simulink model "PI Controller Vector Controlled IM Drive"  (R2020b)
settings: Solver=ode4  StartTime=0.0  StopTime=5  RelTol=1e-3
InitFcn:
  | %clear;
  | %clc;
  | 
  | %Motor Parameters
  | r1 = 1.405;
  | l1  = 0.005839;
  | r2 = 1.395;
  | l2 = 0.005839;
  | Lm = 0.1722;
  | J = 0.0131;
  | 
  | %Motor Rated Values
  | Vrat = 400;
  | frat = 50;
  | 
  | x1 = 2*pi*frat*l1;
  | x2 = 2*pi*frat*l2;
  | Xm = 2*pi*frat*Lm;
  | Prat = 4*1000;
  | Nrat = 1430;
  | P = 4;
  | Ns = 120*frat/P;
  | nrat = Nrat*2*pi/60;
  | ns = Ns*2*pi/60;
  | srat = (Ns-Nrat)/Ns;
  | 
  | E1 = Vrat/sqrt(3); %phase voltage
  | IL = E1/( (r1 + (1i*x1) ) + ( ( (1i*x2) +(r2/srat) )*1i*Xm / ( (1i*Xm) + (1i*x2) + (r2/srat) ) ) );
  | E2 = E1 - (IL*(r1 + (1i*x1) ) );
  | Trat = (3/(ns))*srat*abs(E2)*abs(E2)*r2/((r2*r2) + (srat*srat*x2*x2));
  | %Trat = Prat/nrat;
  | 
  | %System Variables
  | Tsys = (1e-6);
  | Ts = (100e-6);
  | freq = 50;
  | ws = freq*2*pi;
  | 
  | m=1*freq/50;
  | %m = 1 * (freq/50);
  | Vbus = (400*sqrt(2)*2/sqrt(3)) / (1.15);
  | 
  | Vref = (Vbus*sqrt(3)/2) * m;
  | delay = Ts/Tsys;
  | 
  | % Motor Starting Parameters
  | inc_time = 0.1;
  | 
  | %Motor Loading time
  | load_time = 0;
  | 
  | %No. of Hybrid Zones
  | numzones = 3;
  | 
  | %Load ML model Weights
  | 
  | W1R_s1 = readmatrix('Regression Weights\W1_subnet1_tmp_odd_90.xlsx');
  | b1R_s1 = readmatrix('Regression Weights\b1_subnet1_tmp_odd_90.xlsx');
  | W1R_s2 = readmatrix('Regression Weights\W1_subnet2_tmp_odd_90.xlsx');
  | b1R_s2 = readmatrix('Regression Weights\b1_subnet2_tmp_odd_90.xlsx');
  | ... (+35 lines)
undefined symbols (not defined in the file): DiscIntNeverNeededParam
libraries: powerlib x21, simulink x19, pid_lib x4, powerlib_meascontrol x4, simulink_extras x2
(part 2 of 3)

== system PI Controller Vector Controlled IM Drive/Space Vector PWM based VSI 1/Gating Pulse Generator/Gate Pulse Generator for 2721 Sequence ==
  "S1, S3, S5, sector" : Inport
  AND{,1..5} (6 alike) : Logic  IconShape=distinctive  AllPortsSameDT=off  OutDataTypeStr=boolean
  Constant : Constant  Value=2
  Data Type Conversion : DataTypeConversion
  Demux : Demux
  For Even Sector : Subsystem
  For Odd Sector : Subsystem
  Mod : Math  Operator=mod  SaturateOnIntegerOverflow=on
  Mux : Mux  Inputs=3
  NOT : Logic  Operator=NOT  IconShape=distinctive  AllPortsSameDT=off  OutDataTypeStr=boolean
  OR : Logic  Operator=OR  IconShape=distinctive  AllPortsSameDT=off  OutDataTypeStr=boolean
  OR1 : Logic  Operator=OR  IconShape=distinctive  AllPortsSameDT=off  OutDataTypeStr=boolean
  OR2 : Logic  Operator=OR  IconShape=distinctive  AllPortsSameDT=off  OutDataTypeStr=boolean
  Scope1 : Scope  NumInputPorts=4
  Gate 1 Pulse : Outport
  Gate 3 Pulse : Outport  Port=2
  Gate 5 Pulse : Outport  Port=3
  wires:
  For Odd Sector/3(Gate 5 Pulse) -> AND5/1
  For Odd Sector/1(Gate 1 Pulse) -> AND3/1
  For Even Sector/3(Gate 5 Pulse) -> AND2/1
  OR2/1 -> Scope1/3, Gate 5 Pulse/1
  For Even Sector/2(Gate 3 Pulse) -> AND1/1
  OR1/1 -> Scope1/2, Gate 3 Pulse/1
  Demux/3 -> Mux/3
  AND4/1 -> OR1/1
  OR/1 -> Scope1/1, Gate 1 Pulse/1
  AND5/1 -> OR2/1
  Demux/2 -> Mux/2
  For Odd Sector/2(Gate 3 Pulse) -> AND4/1
  AND1/1 -> OR1/2
  AND/1 -> OR/2
  Mod/1 -> Data Type Conversion/1
  Data Type Conversion/1 -> AND3/2, AND4/2, AND5/2, NOT/1
  AND2/1 -> OR2/2
  "S1, S3, S5, sector"/1 -> Demux/1
  AND3/1 -> OR/1
  Demux/4 -> Scope1/4, Mod/1
  Demux/1 -> Mux/1
  Mux/1 -> For Even Sector/1("S1, S3, S5"), For Odd Sector/1("S1, S3, S1")
  Constant/1 -> Mod/2
  NOT/1 -> AND/2, AND1/2, AND2/2
  For Even Sector/1(Gate 1 Pulse) -> AND/1

== system PI Controller Vector Controlled IM Drive/Space Vector PWM based VSI 1/Gating Pulse Generator/Gate Pulse Generator for 7212 Sequence ==
  "S1, S3, S5, sector" : Inport
  AND{,1..5} (6 alike) : Logic  IconShape=distinctive  AllPortsSameDT=off  OutDataTypeStr=boolean
  Constant : Constant  Value=2
  Data Type Conversion : DataTypeConversion
  Demux : Demux
  For Even Sector : Subsystem
  For Odd Sector : Subsystem
  Mod : Math  Operator=mod  SaturateOnIntegerOverflow=on
  Mux : Mux  Inputs=3
  NOT : Logic  Operator=NOT  IconShape=distinctive  AllPortsSameDT=off  OutDataTypeStr=boolean
  OR : Logic  Operator=OR  IconShape=distinctive  AllPortsSameDT=off  OutDataTypeStr=boolean
  OR1 : Logic  Operator=OR  IconShape=distinctive  AllPortsSameDT=off  OutDataTypeStr=boolean
  OR2 : Logic  Operator=OR  IconShape=distinctive  AllPortsSameDT=off  OutDataTypeStr=boolean
  Scope1 : Scope  NumInputPorts=4
  Gate 1 Pulse : Outport
  Gate 3 Pulse : Outport  Port=2
  Gate 5 Pulse : Outport  Port=3
  wires:
  For Odd Sector/3(Gate 5 Pulse) -> AND5/1
  For Odd Sector/1(Gate 1 Pulse) -> AND3/1
  For Even Sector/3(Gate 5 Pulse) -> AND2/1
  For Even Sector/2(Gate 3 Pulse) -> AND1/1
  OR2/1 -> Scope1/3, Gate 5 Pulse/1
  OR1/1 -> Scope1/2, Gate 3 Pulse/1
  Demux/3 -> Mux/3
  For Even Sector/1(Gate 1 Pulse) -> AND/1
  AND4/1 -> OR1/1
  OR/1 -> Scope1/1, Gate 1 Pulse/1
  AND5/1 -> OR2/1
  Demux/2 -> Mux/2
  AND1/1 -> OR1/2
  AND/1 -> OR/2
  Mod/1 -> Data Type Conversion/1
  Demux/4 -> Scope1/4, Mod/1
  Data Type Conversion/1 -> AND3/2, AND4/2, AND5/2, NOT/1
  AND2/1 -> OR2/2
  Demux/1 -> Mux/1
  Mux/1 -> For Even Sector/1("S1, S3, S1"), For Odd Sector/1("S1, S3, S5")
  Constant/1 -> Mod/2
  NOT/1 -> AND/2, AND1/2, AND2/2
  For Odd Sector/2(Gate 3 Pulse) -> AND4/1
  "S1, S3, S5, sector"/1 -> Demux/1
  AND3/1 -> OR/1

== system PI Controller Vector Controlled IM Drive/Space Vector PWM based VSI 1/Switching Times and Sector/Angle Calculation1 ==
  freq : Inport
  Delay : Delay  DelayLength=1  InitialCondition=0  UseCircularBuffer=on
  Gain1 : Gain  Gain=Tsys
  MATLAB Function : MATLAB Function  TreatAsAtomicUnit=on
  Scope : Scope
  Zero-Order Hold : ZeroOrderHold  SampleTime=Ts
  w : Gain  Gain=2*pi
  Angle : Outport
  tag scope: wt=global
  wires:
  freq/1 -> w/1, Scope/1
  Gain1/1 -> MATLAB Function/2(wTs)
  Zero-Order Hold/1 -> Angle/1
  Delay/1 -> MATLAB Function/1(wold)
  MATLAB Function/1(wnew) -> Delay/1, Zero-Order Hold/1, [wt]
  w/1 -> Gain1/1

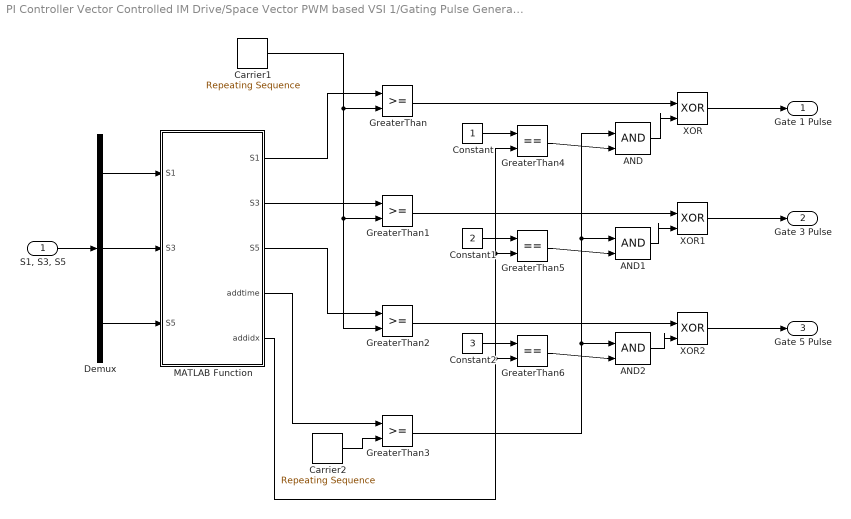
== system PI Controller Vector Controlled IM Drive/Space Vector PWM based VSI 1/Gating Pulse Generator/Gate Pulse Generator for 0121 Sequence/For Even Sector ==
  "S1, S3, S5" : Inport
  AND : Logic  IconShape=distinctive  AllPortsSameDT=off  OutDataTypeStr=boolean
  AND1 : Logic  IconShape=distinctive  AllPortsSameDT=off  OutDataTypeStr=boolean
  AND2 : Logic  IconShape=distinctive  AllPortsSameDT=off  OutDataTypeStr=boolean
  Carrier1 : simulink/Sources/Repeating Sequence  rep_seq_t=[0 Ts/2 Ts]  rep_seq_y=[0 Ts-(1e-16) 0]
  Carrier2 : simulink/Sources/Repeating Sequence  rep_seq_t=[0 Ts/2 Ts]  rep_seq_y=[Ts-(1e-16) 0 Ts-(1e-16)]
  Constant : Constant
  Constant1 : Constant  Value=2
  Constant2 : Constant  Value=3
  Demux : Demux  Outputs=3
  GreaterThan{,1..3} (4 alike) : RelationalOperator  OutDataTypeStr=boolean  RndMeth=Simplest
  GreaterThan4 : RelationalOperator  Operator===  OutDataTypeStr=boolean  RndMeth=Simplest
  GreaterThan5 : RelationalOperator  Operator===  OutDataTypeStr=boolean  RndMeth=Simplest
  GreaterThan6 : RelationalOperator  Operator===  OutDataTypeStr=boolean  RndMeth=Simplest
  MATLAB Function : MATLAB Function  TreatAsAtomicUnit=on
  XOR : Logic  Operator=XOR  IconShape=distinctive  AllPortsSameDT=off  OutDataTypeStr=boolean
  XOR1 : Logic  Operator=XOR  IconShape=distinctive  AllPortsSameDT=off  OutDataTypeStr=boolean
  XOR2 : Logic  Operator=XOR  IconShape=distinctive  AllPortsSameDT=off  OutDataTypeStr=boolean
  Gate 1 Pulse : Outport
  Gate 3 Pulse : Outport  Port=2
  Gate 5 Pulse : Outport  Port=3
  wires:
  Demux/3 -> MATLAB Function/3("S5 ")
  Demux/1 -> MATLAB Function/1("S1 ")
  "S1, S3, S5"/1 -> Demux/1
  Demux/2 -> MATLAB Function/2("S3 ")
  MATLAB Function/5(addidx) -> GreaterThan6/2, GreaterThan5/2, GreaterThan4/2
  Constant1/1 -> GreaterThan5/1
  Constant/1 -> GreaterThan4/1
  XOR1/1 -> Gate 3 Pulse/1
  GreaterThan6/1 -> AND2/2
  Constant2/1 -> GreaterThan6/1
  GreaterThan5/1 -> AND1/2
  AND/1 -> XOR/2
  AND2/1 -> XOR2/2
  GreaterThan2/1 -> XOR2/1
  MATLAB Function/1(S1) -> GreaterThan/1
  GreaterThan/1 -> XOR/1
  MATLAB Function/4(addtime) -> GreaterThan3/1
  GreaterThan4/1 -> AND/2
  XOR2/1 -> Gate 5 Pulse/1
  GreaterThan3/1 -> AND/1, AND1/1, AND2/1
  AND1/1 -> XOR1/2
  MATLAB Function/3(S5) -> GreaterThan2/1
  MATLAB Function/2(S3) -> GreaterThan1/1
  XOR/1 -> Gate 1 Pulse/1
  Carrier1/1 -> GreaterThan/2, GreaterThan1/2, GreaterThan2/2
  GreaterThan1/1 -> XOR1/1
  Carrier2/1 -> GreaterThan3/2

== system PI Controller Vector Controlled IM Drive/Space Vector PWM based VSI 1/Gating Pulse Generator/Gate Pulse Generator for 0121 Sequence/For Odd Sector ==
  "S1, S3, S5" : Inport
  AND : Logic  IconShape=distinctive  AllPortsSameDT=off  OutDataTypeStr=boolean
  AND1 : Logic  IconShape=distinctive  AllPortsSameDT=off  OutDataTypeStr=boolean
  AND2 : Logic  IconShape=distinctive  AllPortsSameDT=off  OutDataTypeStr=boolean
  Carrier1 : simulink/Sources/Repeating Sequence  rep_seq_t=[0 Ts/2 Ts]  rep_seq_y=[Ts-(1e-16) 0 Ts-(1e-16)]
  Constant : Constant
  Constant1 : Constant  Value=2
  Constant2 : Constant  Value=3
  Demux : Demux  Outputs=3
  GreaterThan{,1..3} (4 alike) : RelationalOperator  OutDataTypeStr=boolean  RndMeth=Simplest
  GreaterThan4 : RelationalOperator  Operator===  OutDataTypeStr=boolean  RndMeth=Simplest
  GreaterThan5 : RelationalOperator  Operator===  OutDataTypeStr=boolean  RndMeth=Simplest
  GreaterThan6 : RelationalOperator  Operator===  OutDataTypeStr=boolean  RndMeth=Simplest
  MATLAB Function : MATLAB Function  TreatAsAtomicUnit=on
  XOR : Logic  Operator=XOR  IconShape=distinctive  AllPortsSameDT=off  OutDataTypeStr=boolean
  XOR1 : Logic  Operator=XOR  IconShape=distinctive  AllPortsSameDT=off  OutDataTypeStr=boolean
  XOR2 : Logic  Operator=XOR  IconShape=distinctive  AllPortsSameDT=off  OutDataTypeStr=boolean
  Gate 1 Pulse : Outport
  Gate 3 Pulse : Outport  Port=2
  Gate 5 Pulse : Outport  Port=3
  wires:
  "S1, S3, S5"/1 -> Demux/1
  Demux/1 -> MATLAB Function/1("S1 ")
  Demux/2 -> MATLAB Function/2("S3 ")
  Demux/3 -> MATLAB Function/3("S5 ")
  MATLAB Function/1(S1) -> GreaterThan/1
  Carrier1/1 -> GreaterThan/2, GreaterThan1/2, GreaterThan3/2, GreaterThan2/2
  MATLAB Function/2(S3) -> GreaterThan1/1
  MATLAB Function/3(S5) -> GreaterThan2/1
  MATLAB Function/4(subtime) -> GreaterThan3/1
  MATLAB Function/5(subidx) -> GreaterThan6/2, GreaterThan5/2, GreaterThan4/2
  Constant/1 -> GreaterThan4/1
  Constant1/1 -> GreaterThan5/1
  Constant2/1 -> GreaterThan6/1
  GreaterThan4/1 -> AND/2
  GreaterThan5/1 -> AND1/2
  GreaterThan6/1 -> AND2/2
  GreaterThan3/1 -> AND/1, AND1/1, AND2/1
  AND/1 -> XOR/2
  GreaterThan/1 -> XOR/1
  GreaterThan1/1 -> XOR1/1
  AND1/1 -> XOR1/2
  GreaterThan2/1 -> XOR2/1
  AND2/1 -> XOR2/2
  XOR/1 -> Gate 1 Pulse/1
  XOR1/1 -> Gate 3 Pulse/1
  XOR2/1 -> Gate 5 Pulse/1

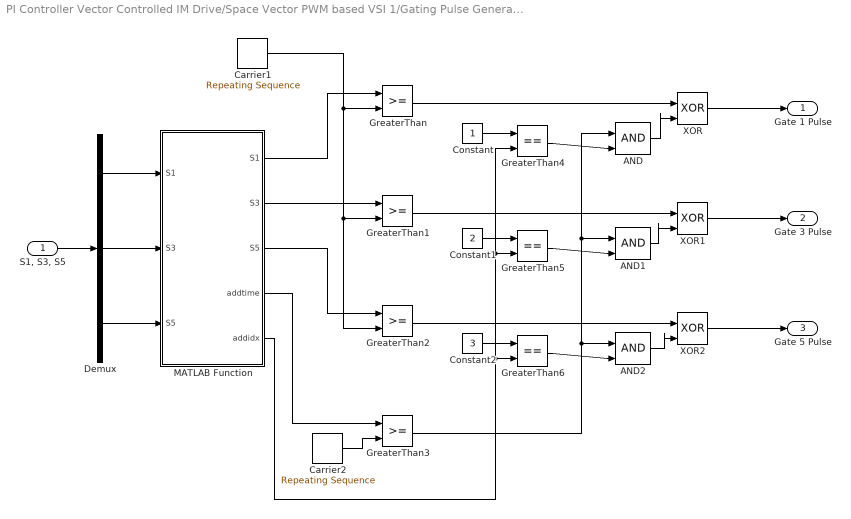
== system PI Controller Vector Controlled IM Drive/Space Vector PWM based VSI 1/Gating Pulse Generator/Gate Pulse Generator for 0127 Sequence 1/For Even Sector ==
  "S1, S3, S5" : Inport
  AND : Logic  IconShape=distinctive  AllPortsSameDT=off  OutDataTypeStr=boolean
  AND1 : Logic  IconShape=distinctive  AllPortsSameDT=off  OutDataTypeStr=boolean
  AND2 : Logic  IconShape=distinctive  AllPortsSameDT=off  OutDataTypeStr=boolean
  Carrier1 : simulink/Sources/Repeating Sequence  rep_seq_t=[0 Ts/2 Ts]  rep_seq_y=[Ts-(1e-16) 0 Ts-(1e-16)]
  Carrier2 : simulink/Sources/Repeating Sequence  rep_seq_t=[0 Ts/2 Ts]  rep_seq_y=[0 Ts-(1e-16) 0]
  Constant : Constant
  Constant1 : Constant  Value=2
  Constant2 : Constant  Value=3
  Demux : Demux  Outputs=3
  GreaterThan{,1..3} (4 alike) : RelationalOperator  OutDataTypeStr=boolean  RndMeth=Simplest
  GreaterThan4 : RelationalOperator  Operator===  OutDataTypeStr=boolean  RndMeth=Simplest
  GreaterThan5 : RelationalOperator  Operator===  OutDataTypeStr=boolean  RndMeth=Simplest
  GreaterThan6 : RelationalOperator  Operator===  OutDataTypeStr=boolean  RndMeth=Simplest
  MATLAB Function : MATLAB Function  TreatAsAtomicUnit=on
  XOR : Logic  Operator=XOR  IconShape=distinctive  AllPortsSameDT=off  OutDataTypeStr=boolean
  XOR1 : Logic  Operator=XOR  IconShape=distinctive  AllPortsSameDT=off  OutDataTypeStr=boolean
  XOR2 : Logic  Operator=XOR  IconShape=distinctive  AllPortsSameDT=off  OutDataTypeStr=boolean
  Gate 1 Pulse : Outport
  Gate 3 Pulse : Outport  Port=2
  Gate 5 Pulse : Outport  Port=3
  wires:
  AND/1 -> XOR/2
  GreaterThan2/1 -> XOR2/1
  "S1, S3, S5"/1 -> Demux/1
  MATLAB Function/1(S1) -> GreaterThan/1
  Demux/1 -> MATLAB Function/1("S1 ")
  Demux/2 -> MATLAB Function/2("S3 ")
  Demux/3 -> MATLAB Function/3("S5 ")
  Carrier2/1 -> GreaterThan3/2
  XOR2/1 -> Gate 5 Pulse/1
  GreaterThan6/1 -> AND2/2
  GreaterThan1/1 -> XOR1/1
  GreaterThan3/1 -> AND/1, AND1/1, AND2/1
  GreaterThan4/1 -> AND/2
  Constant2/1 -> GreaterThan6/1
  AND1/1 -> XOR1/2
  MATLAB Function/2(S3) -> GreaterThan1/1
  MATLAB Function/4(addtime) -> GreaterThan3/1
  XOR/1 -> Gate 1 Pulse/1
  Carrier1/1 -> GreaterThan/2, GreaterThan1/2, GreaterThan2/2
  Constant/1 -> GreaterThan4/1
  MATLAB Function/5(addidx) -> GreaterThan6/2, GreaterThan5/2, GreaterThan4/2
  GreaterThan5/1 -> AND1/2
  GreaterThan/1 -> XOR/1
  XOR1/1 -> Gate 3 Pulse/1
  MATLAB Function/3(S5) -> GreaterThan2/1
  AND2/1 -> XOR2/2
  Constant1/1 -> GreaterThan5/1

== system PI Controller Vector Controlled IM Drive/Space Vector PWM based VSI 1/Gating Pulse Generator/Gate Pulse Generator for 0127 Sequence 1/For Odd Sector ==
  "S1, S3, S1" : Inport
  AND3 : Logic  IconShape=distinctive  AllPortsSameDT=off  OutDataTypeStr=boolean
  AND4 : Logic  IconShape=distinctive  AllPortsSameDT=off  OutDataTypeStr=boolean
  AND5 : Logic  IconShape=distinctive  AllPortsSameDT=off  OutDataTypeStr=boolean
  Carrier3 : simulink/Sources/Repeating Sequence  rep_seq_t=[0 Ts/2 Ts]  rep_seq_y=[0 Ts-(1e-16) 0]
  Constant3 : Constant
  Constant4 : Constant  Value=2
  Constant5 : Constant  Value=3
  Demux1 : Demux  Outputs=3
  GreaterThan{7..10} (4 alike) : RelationalOperator  OutDataTypeStr=boolean  RndMeth=Simplest
  GreaterThan11 : RelationalOperator  Operator===  OutDataTypeStr=boolean  RndMeth=Simplest
  GreaterThan12 : RelationalOperator  Operator===  OutDataTypeStr=boolean  RndMeth=Simplest
  GreaterThan13 : RelationalOperator  Operator===  OutDataTypeStr=boolean  RndMeth=Simplest
  MATLAB Function1 : MATLAB Function  TreatAsAtomicUnit=on
  XOR3 : Logic  Operator=XOR  IconShape=distinctive  AllPortsSameDT=off  OutDataTypeStr=boolean
  XOR4 : Logic  Operator=XOR  IconShape=distinctive  AllPortsSameDT=off  OutDataTypeStr=boolean
  XOR5 : Logic  Operator=XOR  IconShape=distinctive  AllPortsSameDT=off  OutDataTypeStr=boolean
  Gate 1 Pulse1 : Outport
  Gate 3 Pulse1 : Outport  Port=2
  Gate 5 Pulse1 : Outport  Port=3
  wires:
  GreaterThan12/1 -> AND4/2
  GreaterThan9/1 -> XOR5/1
  Constant4/1 -> GreaterThan12/1
  MATLAB Function1/3(S5) -> GreaterThan9/1
  GreaterThan10/1 -> AND3/1, AND4/1, AND5/1
  MATLAB Function1/5(subidx) -> GreaterThan13/2, GreaterThan12/2, GreaterThan11/2
  MATLAB Function1/2(S3) -> GreaterThan8/1
  AND5/1 -> XOR5/2
  Demux1/2 -> MATLAB Function1/2("S3 ")
  AND4/1 -> XOR4/2
  Demux1/1 -> MATLAB Function1/1("S1 ")
  GreaterThan11/1 -> AND3/2
  AND3/1 -> XOR3/2
  MATLAB Function1/1(S1) -> GreaterThan7/1
  GreaterThan8/1 -> XOR4/1
  GreaterThan13/1 -> AND5/2
  Constant5/1 -> GreaterThan13/1
  GreaterThan7/1 -> XOR3/1
  XOR4/1 -> Gate 3 Pulse1/1
  Demux1/3 -> MATLAB Function1/3("S5 ")
  XOR5/1 -> Gate 5 Pulse1/1
  Constant3/1 -> GreaterThan11/1
  XOR3/1 -> Gate 1 Pulse1/1
  "S1, S3, S1"/1 -> Demux1/1
  Carrier3/1 -> GreaterThan7/2, GreaterThan8/2, GreaterThan10/2, GreaterThan9/2
  MATLAB Function1/4(subtime) -> GreaterThan10/1

== system PI Controller Vector Controlled IM Drive/Space Vector PWM based VSI 1/Gating Pulse Generator/Gate Pulse Generator for 1012 Sequence/For Even Sector ==
  "S1, S3, S1" : Inport
  AND3 : Logic  IconShape=distinctive  AllPortsSameDT=off  OutDataTypeStr=boolean
  AND4 : Logic  IconShape=distinctive  AllPortsSameDT=off  OutDataTypeStr=boolean
  AND5 : Logic  IconShape=distinctive  AllPortsSameDT=off  OutDataTypeStr=boolean
  Carrier2 : simulink/Sources/Repeating Sequence  rep_seq_t=[0 Ts/2 Ts]  rep_seq_y=[0 Ts-(1e-16) 0]
  Constant3 : Constant
  Constant4 : Constant  Value=2
  Constant5 : Constant  Value=3
  Demux1 : Demux  Outputs=3
  GreaterThan{7..10} (4 alike) : RelationalOperator  OutDataTypeStr=boolean  RndMeth=Simplest
  GreaterThan11 : RelationalOperator  Operator===  OutDataTypeStr=boolean  RndMeth=Simplest
  GreaterThan12 : RelationalOperator  Operator===  OutDataTypeStr=boolean  RndMeth=Simplest
  GreaterThan13 : RelationalOperator  Operator===  OutDataTypeStr=boolean  RndMeth=Simplest
  MATLAB Function1 : MATLAB Function  TreatAsAtomicUnit=on
  XOR3 : Logic  Operator=XOR  IconShape=distinctive  AllPortsSameDT=off  OutDataTypeStr=boolean
  XOR4 : Logic  Operator=XOR  IconShape=distinctive  AllPortsSameDT=off  OutDataTypeStr=boolean
  XOR5 : Logic  Operator=XOR  IconShape=distinctive  AllPortsSameDT=off  OutDataTypeStr=boolean
  Gate 1 Pulse : Outport
  Gate 3 Pulse : Outport  Port=2
  Gate 5 Pulse : Outport  Port=3
  wires:
  XOR3/1 -> Gate 1 Pulse/1
  XOR5/1 -> Gate 5 Pulse/1
  Demux1/3 -> MATLAB Function1/3("S5 ")
  GreaterThan7/1 -> XOR3/1
  GreaterThan11/1 -> AND3/2
  Demux1/2 -> MATLAB Function1/2("S3 ")
  GreaterThan8/1 -> XOR4/1
  XOR4/1 -> Gate 3 Pulse/1
  AND4/1 -> XOR4/2
  AND3/1 -> XOR3/2
  MATLAB Function1/4(subtime) -> GreaterThan10/1
  AND5/1 -> XOR5/2
  GreaterThan13/1 -> AND5/2
  Constant5/1 -> GreaterThan13/1
  Constant3/1 -> GreaterThan11/1
  MATLAB Function1/2(S3) -> GreaterThan8/1
  Demux1/1 -> MATLAB Function1/1("S1 ")
  MATLAB Function1/5(subidx) -> GreaterThan13/2, GreaterThan12/2, GreaterThan11/2
  MATLAB Function1/3(S5) -> GreaterThan9/1
  MATLAB Function1/1(S1) -> GreaterThan7/1
  GreaterThan10/1 -> AND3/1, AND4/1, AND5/1
  Constant4/1 -> GreaterThan12/1
  GreaterThan9/1 -> XOR5/1
  "S1, S3, S1"/1 -> Demux1/1
  Carrier2/1 -> GreaterThan7/2, GreaterThan8/2, GreaterThan10/2, GreaterThan9/2
  GreaterThan12/1 -> AND4/2

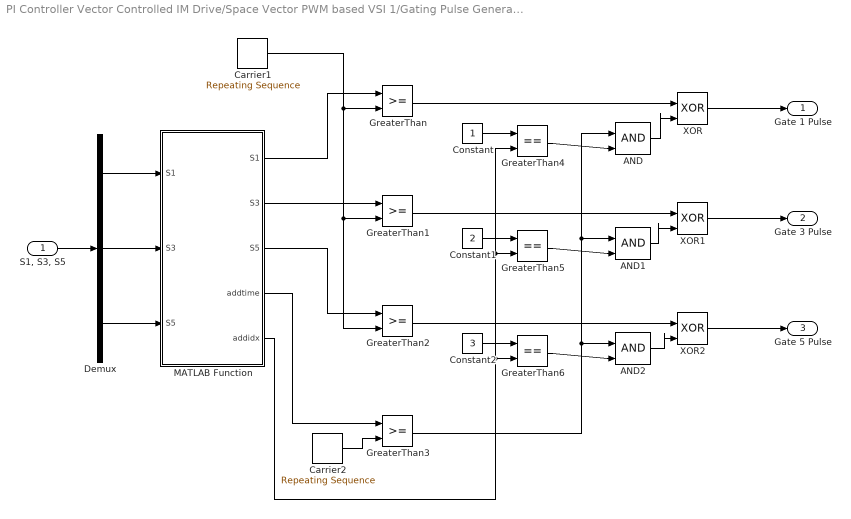
== system PI Controller Vector Controlled IM Drive/Space Vector PWM based VSI 1/Gating Pulse Generator/Gate Pulse Generator for 1012 Sequence/For Odd Sector ==
  "S1, S3, S5" : Inport
  AND : Logic  IconShape=distinctive  AllPortsSameDT=off  OutDataTypeStr=boolean
  AND1 : Logic  IconShape=distinctive  AllPortsSameDT=off  OutDataTypeStr=boolean
  AND2 : Logic  IconShape=distinctive  AllPortsSameDT=off  OutDataTypeStr=boolean
  Carrier1 : simulink/Sources/Repeating Sequence  rep_seq_t=[0 Ts/2 Ts]  rep_seq_y=[Ts-(1e-16) 0 Ts-(1e-16)]
  Carrier2 : simulink/Sources/Repeating Sequence  rep_seq_t=[0 Ts/2 Ts]  rep_seq_y=[0 Ts-(1e-16) 0]
  Constant : Constant
  Constant1 : Constant  Value=2
  Constant2 : Constant  Value=3
  Demux : Demux  Outputs=3
  GreaterThan{,1..3} (4 alike) : RelationalOperator  OutDataTypeStr=boolean  RndMeth=Simplest
  GreaterThan4 : RelationalOperator  Operator===  OutDataTypeStr=boolean  RndMeth=Simplest
  GreaterThan5 : RelationalOperator  Operator===  OutDataTypeStr=boolean  RndMeth=Simplest
  GreaterThan6 : RelationalOperator  Operator===  OutDataTypeStr=boolean  RndMeth=Simplest
  MATLAB Function : MATLAB Function  TreatAsAtomicUnit=on
  XOR : Logic  Operator=XOR  IconShape=distinctive  AllPortsSameDT=off  OutDataTypeStr=boolean
  XOR1 : Logic  Operator=XOR  IconShape=distinctive  AllPortsSameDT=off  OutDataTypeStr=boolean
  XOR2 : Logic  Operator=XOR  IconShape=distinctive  AllPortsSameDT=off  OutDataTypeStr=boolean
  Gate 1 Pulse : Outport
  Gate 3 Pulse : Outport  Port=2
  Gate 5 Pulse : Outport  Port=3
  wires:
  Carrier1/1 -> GreaterThan/2, GreaterThan1/2, GreaterThan2/2
  MATLAB Function/2(S3) -> GreaterThan1/1
  XOR/1 -> Gate 1 Pulse/1
  MATLAB Function/3(S5) -> GreaterThan2/1
  Constant/1 -> GreaterThan4/1
  MATLAB Function/4(addtime) -> GreaterThan3/1
  GreaterThan/1 -> XOR/1
  AND1/1 -> XOR1/2
  GreaterThan3/1 -> AND/1, AND1/1, AND2/1
  GreaterThan1/1 -> XOR1/1
  XOR2/1 -> Gate 5 Pulse/1
  GreaterThan4/1 -> AND/2
  MATLAB Function/1(S1) -> GreaterThan/1
  Carrier2/1 -> GreaterThan3/2
  GreaterThan2/1 -> XOR2/1
  GreaterThan5/1 -> AND1/2
  Constant2/1 -> GreaterThan6/1
  "S1, S3, S5"/1 -> Demux/1
  AND/1 -> XOR/2
  AND2/1 -> XOR2/2
  Constant1/1 -> GreaterThan5/1
  XOR1/1 -> Gate 3 Pulse/1
  MATLAB Function/5(addidx) -> GreaterThan6/2, GreaterThan5/2, GreaterThan4/2
  Demux/3 -> MATLAB Function/3("S5 ")
  Demux/1 -> MATLAB Function/1("S1 ")
  Demux/2 -> MATLAB Function/2("S3 ")
  GreaterThan6/1 -> AND2/2

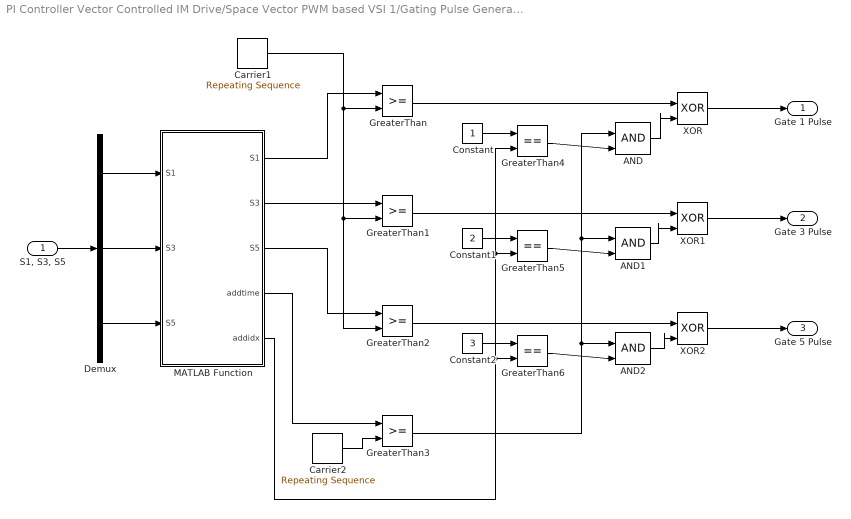
== system PI Controller Vector Controlled IM Drive/Space Vector PWM based VSI 1/Gating Pulse Generator/Gate Pulse Generator for 2721 Sequence/For Even Sector ==
  "S1, S3, S5" : Inport
  AND : Logic  IconShape=distinctive  AllPortsSameDT=off  OutDataTypeStr=boolean
  AND1 : Logic  IconShape=distinctive  AllPortsSameDT=off  OutDataTypeStr=boolean
  AND2 : Logic  IconShape=distinctive  AllPortsSameDT=off  OutDataTypeStr=boolean
  Carrier1 : simulink/Sources/Repeating Sequence  rep_seq_t=[0 Ts/2 Ts]  rep_seq_y=[Ts-(1e-16) 0 Ts-(1e-16)]
  Carrier2 : simulink/Sources/Repeating Sequence  rep_seq_t=[0 Ts/2 Ts]  rep_seq_y=[0 Ts-(1e-16) 0]
  Constant : Constant
  Constant1 : Constant  Value=2
  Constant2 : Constant  Value=3
  Demux : Demux  Outputs=3
  GreaterThan{,1..3} (4 alike) : RelationalOperator  OutDataTypeStr=boolean  RndMeth=Simplest
  GreaterThan4 : RelationalOperator  Operator===  OutDataTypeStr=boolean  RndMeth=Simplest
  GreaterThan5 : RelationalOperator  Operator===  OutDataTypeStr=boolean  RndMeth=Simplest
  GreaterThan6 : RelationalOperator  Operator===  OutDataTypeStr=boolean  RndMeth=Simplest
  MATLAB Function : MATLAB Function  TreatAsAtomicUnit=on
  XOR : Logic  Operator=XOR  IconShape=distinctive  AllPortsSameDT=off  OutDataTypeStr=boolean
  XOR1 : Logic  Operator=XOR  IconShape=distinctive  AllPortsSameDT=off  OutDataTypeStr=boolean
  XOR2 : Logic  Operator=XOR  IconShape=distinctive  AllPortsSameDT=off  OutDataTypeStr=boolean
  Gate 1 Pulse : Outport
  Gate 3 Pulse : Outport  Port=2
  Gate 5 Pulse : Outport  Port=3
  wires:
  AND/1 -> XOR/2
  GreaterThan2/1 -> XOR2/1
  "S1, S3, S5"/1 -> Demux/1
  MATLAB Function/1(S1) -> GreaterThan/1
  Demux/1 -> MATLAB Function/1("S1 ")
  Demux/2 -> MATLAB Function/2("S3 ")
  Demux/3 -> MATLAB Function/3("S5 ")
  Carrier2/1 -> GreaterThan3/2
  XOR2/1 -> Gate 5 Pulse/1
  GreaterThan6/1 -> AND2/2
  GreaterThan1/1 -> XOR1/1
  GreaterThan3/1 -> AND/1, AND1/1, AND2/1
  GreaterThan4/1 -> AND/2
  Constant2/1 -> GreaterThan6/1
  AND1/1 -> XOR1/2
  MATLAB Function/2(S3) -> GreaterThan1/1
  MATLAB Function/4(addtime) -> GreaterThan3/1
  XOR/1 -> Gate 1 Pulse/1
  Carrier1/1 -> GreaterThan/2, GreaterThan1/2, GreaterThan2/2
  Constant/1 -> GreaterThan4/1
  MATLAB Function/5(addidx) -> GreaterThan6/2, GreaterThan5/2, GreaterThan4/2
  GreaterThan5/1 -> AND1/2
  GreaterThan/1 -> XOR/1
  XOR1/1 -> Gate 3 Pulse/1
  MATLAB Function/3(S5) -> GreaterThan2/1
  AND2/1 -> XOR2/2
  Constant1/1 -> GreaterThan5/1

== system PI Controller Vector Controlled IM Drive/Space Vector PWM based VSI 1/Gating Pulse Generator/Gate Pulse Generator for 2721 Sequence/For Odd Sector ==
  "S1, S3, S1" : Inport
  AND3 : Logic  IconShape=distinctive  AllPortsSameDT=off  OutDataTypeStr=boolean
  AND4 : Logic  IconShape=distinctive  AllPortsSameDT=off  OutDataTypeStr=boolean
  AND5 : Logic  IconShape=distinctive  AllPortsSameDT=off  OutDataTypeStr=boolean
  Carrier3 : simulink/Sources/Repeating Sequence  rep_seq_t=[0 Ts/2 Ts]  rep_seq_y=[0 Ts-(1e-16) 0]
  Constant3 : Constant
  Constant4 : Constant  Value=2
  Constant5 : Constant  Value=3
  Demux1 : Demux  Outputs=3
  GreaterThan{7..10} (4 alike) : RelationalOperator  OutDataTypeStr=boolean  RndMeth=Simplest
  GreaterThan11 : RelationalOperator  Operator===  OutDataTypeStr=boolean  RndMeth=Simplest
  GreaterThan12 : RelationalOperator  Operator===  OutDataTypeStr=boolean  RndMeth=Simplest
  GreaterThan13 : RelationalOperator  Operator===  OutDataTypeStr=boolean  RndMeth=Simplest
  MATLAB Function1 : MATLAB Function  TreatAsAtomicUnit=on
  XOR3 : Logic  Operator=XOR  IconShape=distinctive  AllPortsSameDT=off  OutDataTypeStr=boolean
  XOR4 : Logic  Operator=XOR  IconShape=distinctive  AllPortsSameDT=off  OutDataTypeStr=boolean
  XOR5 : Logic  Operator=XOR  IconShape=distinctive  AllPortsSameDT=off  OutDataTypeStr=boolean
  Gate 1 Pulse : Outport
  Gate 3 Pulse : Outport  Port=2
  Gate 5 Pulse : Outport  Port=3
  wires:
  GreaterThan12/1 -> AND4/2
  GreaterThan9/1 -> XOR5/1
  Constant4/1 -> GreaterThan12/1
  MATLAB Function1/3(S5) -> GreaterThan9/1
  GreaterThan10/1 -> AND3/1, AND4/1, AND5/1
  MATLAB Function1/5(subidx) -> GreaterThan13/2, GreaterThan12/2, GreaterThan11/2
  MATLAB Function1/2(S3) -> GreaterThan8/1
  AND5/1 -> XOR5/2
  Demux1/2 -> MATLAB Function1/2("S3 ")
  AND4/1 -> XOR4/2
  Demux1/1 -> MATLAB Function1/1("S1 ")
  GreaterThan11/1 -> AND3/2
  AND3/1 -> XOR3/2
  MATLAB Function1/1(S1) -> GreaterThan7/1
  GreaterThan8/1 -> XOR4/1
  GreaterThan13/1 -> AND5/2
  Constant5/1 -> GreaterThan13/1
  GreaterThan7/1 -> XOR3/1
  XOR4/1 -> Gate 3 Pulse/1
  Demux1/3 -> MATLAB Function1/3("S5 ")
  XOR5/1 -> Gate 5 Pulse/1
  Constant3/1 -> GreaterThan11/1
  XOR3/1 -> Gate 1 Pulse/1
  "S1, S3, S1"/1 -> Demux1/1
  Carrier3/1 -> GreaterThan7/2, GreaterThan8/2, GreaterThan10/2, GreaterThan9/2
  MATLAB Function1/4(subtime) -> GreaterThan10/1

== system PI Controller Vector Controlled IM Drive/Space Vector PWM based VSI 1/Gating Pulse Generator/Gate Pulse Generator for 7212 Sequence/For Even Sector ==
  "S1, S3, S1" : Inport
  AND3 : Logic  IconShape=distinctive  AllPortsSameDT=off  OutDataTypeStr=boolean
  AND4 : Logic  IconShape=distinctive  AllPortsSameDT=off  OutDataTypeStr=boolean
  AND5 : Logic  IconShape=distinctive  AllPortsSameDT=off  OutDataTypeStr=boolean
  Carrier3 : simulink/Sources/Repeating Sequence  rep_seq_t=[0 Ts/2 Ts]  rep_seq_y=[Ts-(1e-16) 0 Ts-(1e-16)]
  Constant3 : Constant
  Constant4 : Constant  Value=2
  Constant5 : Constant  Value=3
  Demux1 : Demux  Outputs=3
  GreaterThan{7..10} (4 alike) : RelationalOperator  OutDataTypeStr=boolean  RndMeth=Simplest
  GreaterThan11 : RelationalOperator  Operator===  OutDataTypeStr=boolean  RndMeth=Simplest
  GreaterThan12 : RelationalOperator  Operator===  OutDataTypeStr=boolean  RndMeth=Simplest
  GreaterThan13 : RelationalOperator  Operator===  OutDataTypeStr=boolean  RndMeth=Simplest
  MATLAB Function1 : MATLAB Function  TreatAsAtomicUnit=on
  XOR3 : Logic  Operator=XOR  IconShape=distinctive  AllPortsSameDT=off  OutDataTypeStr=boolean
  XOR4 : Logic  Operator=XOR  IconShape=distinctive  AllPortsSameDT=off  OutDataTypeStr=boolean
  XOR5 : Logic  Operator=XOR  IconShape=distinctive  AllPortsSameDT=off  OutDataTypeStr=boolean
  Gate 1 Pulse : Outport
  Gate 3 Pulse : Outport  Port=2
  Gate 5 Pulse : Outport  Port=3
  wires:
  XOR3/1 -> Gate 1 Pulse/1
  XOR5/1 -> Gate 5 Pulse/1
  Demux1/3 -> MATLAB Function1/3("S5 ")
  GreaterThan7/1 -> XOR3/1
  GreaterThan11/1 -> AND3/2
  Demux1/2 -> MATLAB Function1/2("S3 ")
  GreaterThan8/1 -> XOR4/1
  XOR4/1 -> Gate 3 Pulse/1
  AND4/1 -> XOR4/2
  AND3/1 -> XOR3/2
  MATLAB Function1/4(subtime) -> GreaterThan10/1
  AND5/1 -> XOR5/2
  GreaterThan13/1 -> AND5/2
  Constant5/1 -> GreaterThan13/1
  Constant3/1 -> GreaterThan11/1
  MATLAB Function1/2(S3) -> GreaterThan8/1
  Demux1/1 -> MATLAB Function1/1("S1 ")
  MATLAB Function1/5(subidx) -> GreaterThan13/2, GreaterThan12/2, GreaterThan11/2
  MATLAB Function1/3(S5) -> GreaterThan9/1
  MATLAB Function1/1(S1) -> GreaterThan7/1
  GreaterThan10/1 -> AND3/1, AND4/1, AND5/1
  Constant4/1 -> GreaterThan12/1
  GreaterThan9/1 -> XOR5/1
  "S1, S3, S1"/1 -> Demux1/1
  Carrier3/1 -> GreaterThan7/2, GreaterThan8/2, GreaterThan10/2, GreaterThan9/2
  GreaterThan12/1 -> AND4/2

== system PI Controller Vector Controlled IM Drive/Space Vector PWM based VSI 1/Gating Pulse Generator/Gate Pulse Generator for 7212 Sequence/For Odd Sector ==
  "S1, S3, S5" : Inport
  AND : Logic  IconShape=distinctive  AllPortsSameDT=off  OutDataTypeStr=boolean
  AND1 : Logic  IconShape=distinctive  AllPortsSameDT=off  OutDataTypeStr=boolean
  AND2 : Logic  IconShape=distinctive  AllPortsSameDT=off  OutDataTypeStr=boolean
  Carrier1 : simulink/Sources/Repeating Sequence  rep_seq_t=[0 Ts/2 Ts]  rep_seq_y=[0 Ts-(1e-16) 0]
  Carrier2 : simulink/Sources/Repeating Sequence  rep_seq_t=[0 Ts/2 Ts]  rep_seq_y=[Ts-(1e-16) 0 Ts-(1e-16)]
  Constant : Constant
  Constant1 : Constant  Value=2
  Constant2 : Constant  Value=3
  Demux : Demux  Outputs=3
  GreaterThan{,1..3} (4 alike) : RelationalOperator  OutDataTypeStr=boolean  RndMeth=Simplest
  GreaterThan4 : RelationalOperator  Operator===  OutDataTypeStr=boolean  RndMeth=Simplest
  GreaterThan5 : RelationalOperator  Operator===  OutDataTypeStr=boolean  RndMeth=Simplest
  GreaterThan6 : RelationalOperator  Operator===  OutDataTypeStr=boolean  RndMeth=Simplest
  MATLAB Function : MATLAB Function  TreatAsAtomicUnit=on
  XOR : Logic  Operator=XOR  IconShape=distinctive  AllPortsSameDT=off  OutDataTypeStr=boolean
  XOR1 : Logic  Operator=XOR  IconShape=distinctive  AllPortsSameDT=off  OutDataTypeStr=boolean
  XOR2 : Logic  Operator=XOR  IconShape=distinctive  AllPortsSameDT=off  OutDataTypeStr=boolean
  Gate 1 Pulse : Outport
  Gate 3 Pulse : Outport  Port=2
  Gate 5 Pulse : Outport  Port=3
  wires:
  Carrier1/1 -> GreaterThan/2, GreaterThan1/2, GreaterThan2/2
  MATLAB Function/2(S3) -> GreaterThan1/1
  XOR/1 -> Gate 1 Pulse/1
  MATLAB Function/3(S5) -> GreaterThan2/1
  Constant/1 -> GreaterThan4/1
  MATLAB Function/4(addtime) -> GreaterThan3/1
  GreaterThan/1 -> XOR/1
  AND1/1 -> XOR1/2
  GreaterThan3/1 -> AND/1, AND1/1, AND2/1
  GreaterThan1/1 -> XOR1/1
  XOR2/1 -> Gate 5 Pulse/1
  GreaterThan4/1 -> AND/2
  MATLAB Function/1(S1) -> GreaterThan/1
  Carrier2/1 -> GreaterThan3/2
  GreaterThan2/1 -> XOR2/1
  GreaterThan5/1 -> AND1/2
  Constant2/1 -> GreaterThan6/1
  "S1, S3, S5"/1 -> Demux/1
  AND/1 -> XOR/2
  AND2/1 -> XOR2/2
  Constant1/1 -> GreaterThan5/1
  XOR1/1 -> Gate 3 Pulse/1
  MATLAB Function/5(addidx) -> GreaterThan6/2, GreaterThan5/2, GreaterThan4/2
  Demux/3 -> MATLAB Function/3("S5 ")
  Demux/1 -> MATLAB Function/1("S1 ")
  Demux/2 -> MATLAB Function/2("S3 ")
  GreaterThan6/1 -> AND2/2

== matlab function PI Controller Vector Controlled IM Drive/Space Vector PWM based VSI 1/Gating Pulse Generator/Gate Pulse Generator for 0127 Sequence 1/For Odd Sector/MATLAB Function1 ==
  data: S1 input; S1 output; S3 input; S5 input; S3 output; S5 output; subtime output; subidx output
function [S1, S3, S5, subtime,subidx] = fcn(S1, S3, S5)
    S = [S1 S3 S5];
    [~, idx] = mink([S1 S3 S5], 3);
    
    subtime = ( ( S(idx(2)) - S(idx(1)) )/2);
    S(idx(1)) = S(idx(1)) + subtime;
    subidx = idx(1);
    
    S1 = S(1);
    S3 = S(2);
    S5 = S(3);
end

== matlab function PI Controller Vector Controlled IM Drive/Space Vector PWM based VSI 1/Gating Pulse Generator/Gate Pulse Generator for 1012 Sequence/For Even Sector/MATLAB Function1 ==
  data: S1 input; S1 output; S3 input; S5 input; S3 output; S5 output; subtime output; subidx output
function [S1, S3, S5, subtime,subidx] = fcn(S1, S3, S5)
    S = [S1 S3 S5];
    [~, idx] = mink([S1 S3 S5], 3);
    
    subtime = ( ( S(idx(2)) - S(idx(1)) )/2);
    S(idx(1)) = S(idx(1)) + subtime;
    subidx = idx(1);
    
    S1 = S(1);
    S3 = S(2);
    S5 = S(3);
end

== matlab function PI Controller Vector Controlled IM Drive/Space Vector PWM based VSI 1/Gating Pulse Generator/Gate Pulse Generator for 1012 Sequence/For Odd Sector/MATLAB Function ==
  data: S1 input; S1 output; S3 input; S5 input; S3 output; S5 output; addtime output; addidx output
function [S1, S3, S5, addtime,addidx] = fcn(S1, S3, S5)
    S = [S1 S3 S5];
    [~, idx] = mink([S1 S3 S5], 3);
    
    addtime = (S(idx(3)) - S(idx(2)))/2;
    addidx = idx(3);
    S(idx(3)) = S(idx(3)) - addtime;
    
    S1 = S(1);
    S3 = S(2);
    S5 = S(3);
end

== matlab function PI Controller Vector Controlled IM Drive/Space Vector PWM based VSI 1/Gating Pulse Generator/Gate Pulse Generator for 2721 Sequence/For Even Sector/MATLAB Function ==
  data: S1 input; S1 output; S3 input; S5 input; S3 output; S5 output; addtime output; addidx output
function [S1, S3, S5, addtime,addidx] = fcn(S1, S3, S5)
    S = [S1 S3 S5];
    [~, idx] = mink([S1 S3 S5], 3);
    
    addtime = (S(idx(3)) - S(idx(2)))/2;
    addidx = idx(3);
    S(idx(3)) = S(idx(3)) - addtime;
    
    S1 = S(1);
    S3 = S(2);
    S5 = S(3);
end

== matlab function PI Controller Vector Controlled IM Drive/Space Vector PWM based VSI 1/Gating Pulse Generator/Gate Pulse Generator for 2721 Sequence/For Odd Sector/MATLAB Function1 ==
  data: S1 input; S1 output; S3 input; S5 input; S3 output; S5 output; subtime output; subidx output
function [S1, S3, S5, subtime,subidx] = fcn(S1, S3, S5)
    S = [S1 S3 S5];
    [~, idx] = mink([S1 S3 S5], 3);
    
    subtime = ( ( S(idx(2)) - S(idx(1)) )/2);
    S(idx(1)) = S(idx(1)) + subtime;
    subidx = idx(1);
    
    S1 = S(1);
    S3 = S(2);
    S5 = S(3);
end

== matlab function PI Controller Vector Controlled IM Drive/Decoupler/MATLAB Function ==
  data: w input; wmr output; imr input; isq input; Tr input
function wmr = fcn(w, imr, isq, Tr)
if imr==0
    wmr=w+(1/Tr);
else
    wmr = w + (isq/(Tr*imr));
end
end

== matlab function PI Controller Vector Controlled IM Drive/Space Vector PWM based VSI 1/Gating Pulse Generator/Gate Pulse Generator for 7212 Sequence/For Even Sector/MATLAB Function1 ==
  data: S1 input; S1 output; S3 input; S5 input; S3 output; S5 output; subtime output; subidx output
function [S1, S3, S5, subtime,subidx] = fcn(S1, S3, S5)
    S = [S1 S3 S5];
    [~, idx] = mink([S1 S3 S5], 3);
    
    S(idx(2)) = (S(idx(2)) + S(idx(3)))/2;
    
    subidx = idx(2);
    subtime = S(idx(3)) - S(idx(2));
    
    S1 = S(1);
    S3 = S(2);
    S5 = S(3);
end

== matlab function PI Controller Vector Controlled IM Drive/Space Vector PWM based VSI 1/Gating Pulse Generator/Gate Pulse Generator for 7212 Sequence/For Odd Sector/MATLAB Function ==
  data: S1 input; S1 output; S3 input; S5 input; S3 output; S5 output; addtime output; addidx output
function [S1, S3, S5, addtime,addidx] = fcn(S1, S3, S5)
    S = [S1 S3 S5];
    [~, idx] = mink([S1 S3 S5], 3);
    
    addtime = (S(idx(2)) - S(idx(1)))/2;
    addidx = idx(2);
    S(idx(2)) = S(idx(2)) - addtime;
    
    S1 = S(1);
    S3 = S(2);
    S5 = S(3);
end

== matlab function PI Controller Vector Controlled IM Drive/Space Vector PWM based VSI 1/MATLAB Function ==
  data: angle input; angle_conv output
function angle_conv = fcn(angle)
    if angle<0
        angle_conv=(2*pi)+angle;
    else
        angle_conv=angle;
    end
%     angle_conv = rem(angle_conv + (time*ws), 2*pi);
end

== matlab function PI Controller Vector Controlled IM Drive/Space Vector PWM based VSI 1/MATLAB Function1 ==
  data: past_time input; pres_time output; gap input
function pres_time = fcn(past_time, gap)
    pres_time = past_time + gap;
end

== matlab function PI Controller Vector Controlled IM Drive/Space Vector PWM based VSI 1/Switching Times and Sector/Angle Calculation1/MATLAB Function ==
  data: wold input; wnew output; wTs input
function wnew = fcn(wold, wTs)
    wnew = rem(wold + wTs, 2*pi);
end

== matlab function PI Controller Vector Controlled IM Drive/Space Vector PWM based VSI 1/Switching Times and Sector/Feature Expand ==
  data: X input; new_X output size=[1 18]
function new_X = fcn(X)
    X = X';
    new_X = zeros(1,18);
    new_X(1, 1) = X(1, 1);
    new_X(1, 2) = X(1, 2);
    
    %Include sinusoidal terms (1st order)
    new_X(1, 3) = sin(X(1, 1));
    new_X(1, 4) = sin(X(1, 2));
    new_X(1, 5) = cos(X(1, 1));
    new_X(1, 6) = cos(X(1, 2));
%     new_X(1, 7) = sin(X(1, 1).*X(1, 2));
%     new_X(1, 8) = cos(X(1, 1).*X(1, 2));
    
%Include 2nd harmonic sinusoidal terms
    new_X(1, 7) = sin(2*X(1, 1));
    new_X(1, 8) = sin(2*X(1, 2));
    new_X(1, 9) = cos(2*X(1, 1));
    new_X(1, 10) = cos(2*X(1, 2));
    
        %Include 3rd harmonic sinusoidal terms
    new_X(1, 11) = sin(3*X(1, 1));
    new_X(1, 12) = sin(3*X(1, 2));
    new_X(1, 13) = cos(3*X(1, 1));
    new_X(1, 14) = cos(3*X(1, 2));
    
    %Include 4th harmonic sinusoidal terms
    new_X(1, 15) = sin(4*X(1, 1));
    new_X(1, 16) = sin(4*X(1, 2));
    new_X(1, 17) = cos(4*X(1, 1));
    new_X(1, 18) = cos(4*X(1, 2));

%     %Include 2nd order terms
%     new_X(:, 3) = X(:, 1).*X(:, 1);
%     new_X(:, 4) = X(:, 1).*X(:, 2);
%     new_X(:, 5) = X(:, 2).*X(:, 2);
    
%     %Include 3rd order terms
%     new_X(:, 6) = X(:, 1).*X(:, 1).*X(:, 1);
%     new_X(:, 7) = X(:, 1).*X(:, 1).*X(:, 2);
%     new_X(:, 8) = X(:, 1).*X(:, 2).*X(:, 2);
%     new_X(:, 9) = X(:, 2).*X(:, 2).*X(:, 2);
%     
%     %Incluce 4th order terms
%     new_X(:, 10) = X(:, 1).*X(:, 1).*X(:, 1).*X(:, 1);
%     new_X(:, 11) = X(:, 1).*X(:, 1).*X(:, 1).*X(:, 2);
%     new_X(:, 12) = X(:, 1).*X(:, 1).*X(:, 2).*X(:, 2);
%     new_X(:, 13) = X(:, 1).*X(:, 2).*X(:, 2).*X(:, 2);
%     new_X(:, 14) = X(:, 2).*X(:, 2).*X(:, 2).*X(:, 2);
%     
%     %Incluce 5th order terms
%     new_X(:, 15) = X(:, 1).*X(:, 1).*X(:, 1).*X(:, 1).*X(:, 1);
%     new_X(:, 16) = X(:, 1).*X(:, 1).*X(:, 1).*X(:, 1).*X(:, 2);
%     new_X(:, 17) = X(:, 1).*X(:, 1).*X(:, 1).*X(:, 2).*X(:, 2);
%     new_X(:, 18) = X(:, 1).*X(:, 1).*X(:, 2).*X(:, 2).*X(:, 2);
%     new_X(:, 19) = X(:, 1).*X(:, 2).*X(:, 2).*X(:, 2).*X(:, 2);
%     new_X(:, 20) = X(:, 2).*X(:, 2).*X(:, 2).*X(:, 2).*X(:, 2);
%     
%     %Incluce 6th order terms
%     new_X(:, 21) = X(:, 1).*X(:, 1).*X(:, 1).*X(:, 1).*X(:, 1).*X(:, 1);
%     new_X(:, 22) = X(:, 1).*X(:, 1).*X(:, 1).*X(:, 1).*X(:, 1).*X(:, 2);
%     new_X(:, 23) = X(:, 1).*X(:, 1).*X(:, 1).*X(:, 1).*X(:, 2).*X(:, 2);
%     new_X(:, 24) = X(:, 1).*X(:, 1).*X(:, 1).*X(:, 2).*X(:, 2).*X(:, 2);
%     new_X(:, 25) = X(:, 1).*X(:, 1).*X(:, 2).*X(:, 2).*X(:, 2).*X(:, 2);
%     new_X(:, 26) = X(:, 1).*X(:, 2).*X(:, 2).*X(:, 2).*X(:, 2).*X(:, 2);
%     new_X(:, 27) = X(:, 2).*X(:, 2).*X(:, 2).*X(:, 2).*X(:, 2).*X(:, 2);
end

== matlab function PI Controller Vector Controlled IM Drive/Space Vector PWM based VSI 1/Switching Times and Sector/Feature Expand1 ==
  data: X input; new_X output size=[1 90]
function new_X = fcn(X)
    X = X';
    new_X = zeros(1,90);
    new_X(1, 1) = X(1, 1);
    new_X(1, 2) = X(1, 2);
    
    %Include sinusoidal terms (1st order)
    new_X(1, 3) = sin(X(1, 1));
    new_X(1, 4) = sin(X(1, 2));
    new_X(1, 5) = cos(X(1, 1));
    new_X(1, 6) = cos(X(1, 2));
%     new_X(1, 7) = sin(X(1, 1).*X(1, 2));
%     new_X(1, 8) = cos(X(1, 1).*X(1, 2));
    
% %Include 2nd harmonic sinusoidal terms
%     new_X(1, 7) = sin(2*X(1, 1));
%     new_X(1, 8) = sin(2*X(1, 2));
%     new_X(1, 9) = cos(2*X(1, 1));
%     new_X(1, 10) = cos(2*X(1, 2));
    
        %Include 3rd harmonic sinusoidal terms
    new_X(1, 7) = sin(3*X(1, 1));
    new_X(1, 8) = sin(3*X(1, 2));
    new_X(1, 9) = cos(3*X(1, 1));
    new_X(1, 10) = cos(3*X(1, 2));
    
%     %Include 4th harmonic sinusoidal terms
%     new_X(1, 15) = sin(4*X(1, 1));
%     new_X(1, 16) = sin(4*X(1, 2));
%     new_X(1, 17) = cos(4*X(1, 1));
%     new_X(1, 18) = cos(4*X(1, 2));
       %Include 5th harmonic sinusoidal terms
    new_X(1, 11) = sin(5*X(1, 1));
    new_X(1, 12) = sin(5*X(1, 2));
    new_X(1, 13) = cos(5*X(1, 1));
    new_X(1, 14) = cos(5*X(1, 2));
    
       %Include 7th harmonic sinusoidal terms
    new_X(1, 15) = sin(7*X(1, 1));
    new_X(1, 16) = sin(7*X(1, 2));
    new_X(1, 17) = cos(7*X(1, 1));
    new_X(1, 18) = cos(7*X(1, 2));
    
       %Include 9th harmonic sinusoidal terms
    new_X(1, 19) = sin(9*X(1, 1));
    new_X(1, 20) = sin(9*X(1, 2));
    new_X(1, 21) = cos(9*X(1, 1));
    new_X(1, 22) = cos(9*X(1, 2));

       %Include 11th harmonic sinusoidal terms
    new_X(1, 23) = sin(11*X(1, 1));
    new_X(1, 24) = sin(11*X(1, 2));
    new_X(1, 25) = cos(11*X(1, 1));
    new_X(1, 26) = cos(11*X(1, 2));
    
         %Include 13th harmonic sinusoidal terms
    new_X(1, 27) = sin(13*X(1, 1));
    new_X(1, 28) = sin(13*X(1, 2));
    new_X(1, 29) = cos(13*X(1, 1));
    new_X(1, 30) = cos(13*X(1, 2));
    
         %Include 15th harmonic sinusoidal terms
    new_X(1, 31) = sin(15*X(1, 1));
    new_X(1, 32) = sin(15*X(1, 2));
    new_X(1, 33) = cos(15*X(1, 1));
    new_X(1, 34) = cos(15*X(1, 2));
    
    %Include 17th harmonic sinusoidal terms
    new_X(1, 35) = sin(17*X(1, 1));
    new_X(1, 36) = sin(17*X(1, 2));
    new_X(1, 37) = cos(17*X(1, 1));
    new_X(1, 38) = cos(17*X(1, 2));
    
    %Include 19th harmonic sinusoidal terms
    new_X(1, 39) = sin(19*X(1, 1));
    new_X(1, 40) = sin(19*X(1, 2));
    new_X(1, 41) = cos(19*X(1, 1));
    new_X(1, 42) = cos(19*X(1, 2));
    
    %Include 21th harmonic sinusoidal terms
    new_X(1, 43) = sin(21*X(1, 1));
    new_X(1, 44) = sin(21*X(1, 2));
    new_X(1, 45) = cos(21*X(1, 1));
    new_X(1, 46) = cos(21*X(1, 2));
    
    %Include 23th harmonic sinusoidal terms
    new_X(1, 47) = sin(23*X(1, 1));
    new_X(1, 48) = sin(23*X(1, 2));
    new_X(1, 49) = cos(23*X(1, 1));
    new_X(1, 50) = cos(23*X(1, 2));

    %Include 25th harmonic sinusoidal terms
    new_X(1, 51) = sin(25*X(1, 1));
    new_X(1, 52) = sin(25*X(1, 2));
    new_X(1, 53) = cos(25*X(1, 1));
    new_X(1, 54) = cos(25*X(1, 2));

%Include 27th harmonic sinusoidal terms
    new_X(1, 55) = sin(27*X(1, 1));
    new_X(1, 56) = sin(27*X(1, 2));
    new_X(1, 57) = cos(27*X(1, 1));
    new_X(1, 58) = cos(27*X(1, 2));
    
%Include 29th harmonic sinusoidal terms
    new_X(1, 59) = sin(29*X(1, 1));
    new_X(1, 60) = sin(29*X(1, 2));
    new_X(1, 61) = cos(29*X(1, 1));
    new_X(1, 62) = cos(29*X(1, 2));

%Include 31th harmonic sinusoidal terms
    new_X(1, 63) = sin(31*X(1, 1));
    new_X(1, 64) = sin(31*X(1, 2));
    new_X(1, 65) = cos(31*X(1, 1));
    new_X(1, 66) = cos(31*X(1, 2));

%Include 33th harmonic sinusoidal terms
    new_X(1, 67) = sin(33*X(1, 1));
    new_X(1, 68) = sin(33*X(1, 2));
    new_X(1, 69) = cos(33*X(1, 1));
    new_X(1, 70) = cos(33*X(1, 2));
    
%Include 35th harmonic sinusoidal terms
    new_X(1, 71) = sin(35*X(1, 1));
    new_X(1, 72) = sin(35*X(1, 2));
    new_X(1, 73) = cos(35*X(1, 1));
    new_X(1, 74) = cos(35*X(1, 2));
    
%Include 37th harmonic sinusoidal terms
    new_X(1, 75) = sin(37*X(1, 1));
    new_X(1, 76) = sin(37*X(1, 2));
    new_X(1, 77) = cos(37*X(1, 1));
    new_X(1, 78) = cos(37*X(1, 2));
    
%Include 39th harmonic sinusoidal terms
    new_X(1, 79) = sin(39*X(1, 1));
    new_X(1, 80) = sin(39*X(1, 2));
    new_X(1, 81) = cos(39*X(1, 1));
    new_X(1, 82) = cos(39*X(1, 2));
    
%Include 41th harmonic sinusoidal terms
    new_X(1, 83) = sin(41*X(1, 1));
    new_X(1, 84) = sin(41*X(1, 2));
    new_X(1, 85) = cos(41*X(1, 1));
    new_X(1, 86) = cos(41*X(1, 2));

%Include 43th harmonic sinusoidal terms
    new_X(1, 87) = sin(43*X(1, 1));
    new_X(1, 88) = sin(43*X(1, 2));
    new_X(1, 89) = cos(43*X(1, 1));
    new_X(1, 90) = cos(43*X(1, 2));
%     %Include 2nd order terms
%     new_X(:, 3) = X(:, 1).*X(:, 1);
%     new_X(:, 4) = X(:, 1).*X(:, 2);
%     new_X(:, 5) = X(:, 2).*X(:, 2);
    
%     %Include 3rd order terms
%     new_X(:, 6) = X(:, 1).*X(:, 1).*X(:, 1);
%     new_X(:, 7) = X(:, 1).*X(:, 1).*X(:, 2);
%     new_X(:, 8) = X(:, 1).*X(:, 2).*X(:, 2);
%     new_X(:, 9) = X(:, 2).*X(:, 2).*X(:, 2);
%     
%     %Incluce 4th order terms
%     new_X(:, 10) = X(:, 1).*X(:, 1).*X(:, 1).*X(:, 1);
%     new_X(:, 11) = X(:, 1).*X(:, 1).*X(:, 1).*X(:, 2);
%     new_X(:, 12) = X(:, 1).*X(:, 1).*X(:, 2).*X(:, 2);
%     new_X(:, 13) = X(:, 1).*X(:, 2).*X(:, 2).*X(:, 2);
%     new_X(:, 14) = X(:, 2).*X(:, 2).*X(:, 2).*X(:, 2);
%     
%     %Incluce 5th order terms
%     new_X(:, 15) = X(:, 1).*X(:, 1).*X(:, 1).*X(:, 1).*X(:, 1);
%     new_X(:, 16) = X(:, 1).*X(:, 1).*X(:, 1).*X(:, 1).*X(:, 2);
%     new_X(:, 17) = X(:, 1).*X(:, 1).*X(:, 1).*X(:, 2).*X(:, 2);
%     new_X(:, 18) = X(:, 1).*X(:, 1).*X(:, 2).*X(:, 2).*X(:, 2);
%     new_X(:, 19) = X(:, 1).*X(:, 2).*X(:, 2).*X(:, 2).*X(:, 2);
%     new_X(:, 20) = X(:, 2).*X(:, 2).*X(:, 2).*X(:, 2).*X(:, 2);
%     
%     %Incluce 6th order terms
%     new_X(:, 21) = X(:, 1).*X(:, 1).*X(:, 1).*X(:, 1).*X(:, 1).*X(:, 1);
%     new_X(:, 22) = X(:, 1).*X(:, 1).*X(:, 1).*X(:, 1).*X(:, 1).*X(:, 2);
%     new_X(:, 23) = X(:, 1).*X(:, 1).*X(:, 1).*X(:, 1).*X(:, 2).*X(:, 2);
%     new_X(:, 24) = X(:, 1).*X(:, 1).*X(:, 1).*X(:, 2).*X(:, 2).*X(:, 2);
%     new_X(:, 25) = X(:, 1).*X(:, 1).*X(:, 2).*X(:, 2).*X(:, 2).*X(:, 2);
%     new_X(:, 26) = X(:, 1).*X(:, 2).*X(:, 2).*X(:, 2).*X(:, 2).*X(:, 2);
%     new_X(:, 27) = X(:, 2).*X(:, 2).*X(:, 2).*X(:, 2).*X(:, 2).*X(:, 2);
end

== matlab function PI Controller Vector Controlled IM Drive/Space Vector PWM based VSI 1/Switching Times and Sector/MATLAB Function ==
  data: u input; y output
function y = fcn(u)
    y = 1./(1+exp(-1*u));
end

== matlab function PI Controller Vector Controlled IM Drive/Space Vector PWM based VSI 1/Switching Times and Sector/MATLAB Function1 ==
  data: u input; S1 output; S3 output; S5 output
function [S1, S3, S5] = fcn(u)
    S1 = u(1);
    S3 = u(2);
    S5 = u(3);
end

== matlab function PI Controller Vector Controlled IM Drive/Space Vector PWM based VSI 1/Switching Times and Sector/MATLAB Function2 ==
  data: Vref input; V_alpha output; angle input; V_beta output
function [V_alpha, V_beta] = fcn(Vref, angle)
    V_alpha = Vref*cos(angle);
    V_beta = Vref*sin(angle);
end

== matlab function PI Controller Vector Controlled IM Drive/Space Vector PWM based VSI 1/Switching Times and Sector/MATLAB Function3 ==
  data: u input; u output
function u = fcn(u)
    u(u<0) = 0;
end

== matlab function PI Controller Vector Controlled IM Drive/3 Phase Induction Machine/MATLAB Function ==
  data: phi input; phir_d output; theta_rf input; phir_q output
function [phir_d, phir_q] = fcn(phi, theta_rf)
    phir_d = phi;
    phir_q = 0;
end

== matlab function PI Controller Vector Controlled IM Drive/Space Vector PWM based VSI 1/Switching Times and Sector/MATLAB Function4 ==
  data: u input; y output
function y = fcn(u)
    [~, y] = max(u);
end
